simulink model "Project_Sim_Thyr"  (R2022b)
settings: Solver=FixedStepAuto  StartTime=0.0  StopTime=10  FixedStep=0.0001  RelTol=1e-3
libraries: spsVoltageMeasurementLib x6, spsThyristorLib x5, spsGroundLib x3, spsSeriesRLCBranchLib x3, spsControlledVoltageSourceLib x2, spsACVoltageSourceLib x1, spsCurrentMeasurementLib x1, spsDCMachineLib x1, spsDiodeLib x1, spsMeanLib x1, spsMosfetLib x1, spsPWMGeneratorDCDCLib x1
settings Model: Creator=Lenovo  LastModifiedBy=Lenovo

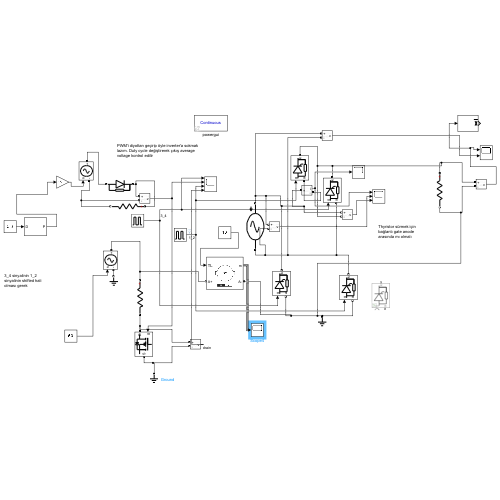
[thumbnail: Simulink's stored preview of the top-level diagram]
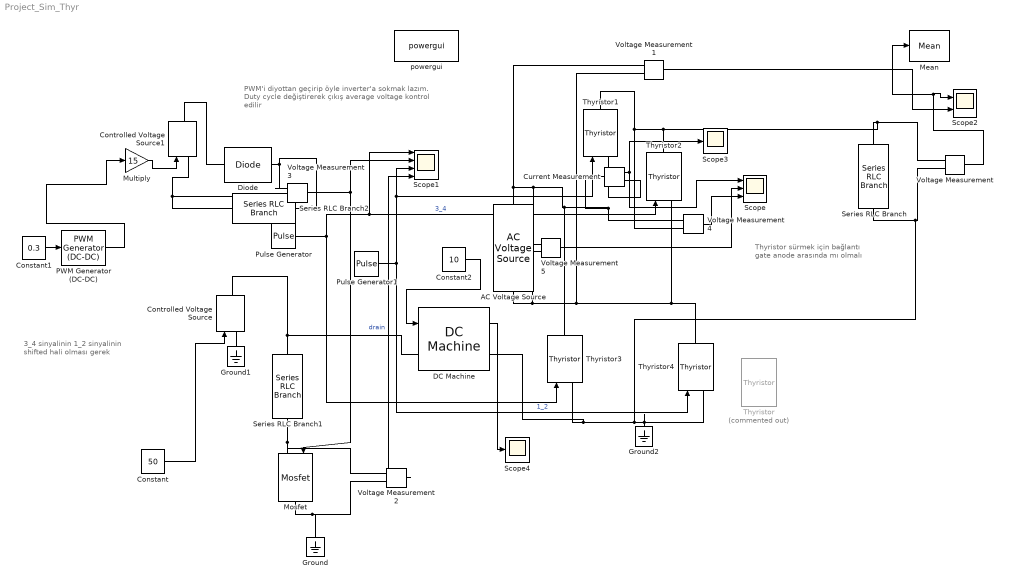
== system Project_Sim_Thyr ==
  note: Thyristor sürmek için bağlantı gate anode arasında mı olmalı
  note: 3_4 sinyalinin 1_2 sinyalinin shifted hali olması gerek
  note: PWM'i diyottan geçirip öyle inverter'a sokmak lazım. Duty cycle değiştirerek çıkış average voltage kontrol edilir
  AC Voltage Source : spsACVoltageSourceLib/AC Voltage Source  Amplitude=230  Phase=0  Frequency=50  SampleTime=0  Measurements=None  BusType=swing  Pref=10e3  Qref=0  Qmin=-inf  Qmax=+inf
  Constant : Constant  Value=50
  Constant1 : Constant  Value=0.3
  Constant2 : Constant  Value=10
  Controlled Voltage Source : spsControlledVoltageSourceLib/Controlled Voltage Source  Initialize=on  Source_Type=DC  Amplitude=15  Phase=0  Frequency=0  Measurements=None
  Controlled Voltage Source1 : spsControlledVoltageSourceLib/Controlled Voltage Source  Initialize=on  Source_Type=DC  Amplitude=0  Phase=0  Frequency=0  Measurements=None
  Current Measurement : spsCurrentMeasurementLib/Current Measurement  PhasorSimulation=off  OutputType=Complex  PSBequivalent=0
  DC Machine : spsDCMachineLib/DC Machine  PresetModel=No  MechanicalLoad=Torque TL  FieldType=Permanent magnet  ShowDetailedParameters=on  MeasurementBus=off  RLa="[ 0.6  0.012]"  RLf="[ 240  120]"  Laf=1.8  MachineConstant=Torque constant (N.m/A)  Ke=1.8  Kt=1.8  J=1  Bm=0  Tf=0  w0=1  Ifinit=1  TsPowergui=0  TsBlock=-1
  Diode : spsDiodeLib/Diode  Ron=0.001  Lon=0  Vf=0.8  IC=0  UseSnubber=0  Rs=500  Cs=250e-9  Measurements=off
  Ground : spsGroundLib/Ground  LConnTagsString=a
  Ground1 : spsGroundLib/Ground  LConnTagsString=a
  Ground2 : spsGroundLib/Ground  LConnTagsString=a
  Mean : spsMeanLib/Mean  Freq=50  Vinit=0  Ts=0
  Mosfet : spsMosfetLib/Mosfet  Ron=0.1  Lon=0  Rd=0.01  Vfd=1  IC=0  Rs=1e5  Cs=inf  Measurements=off
  Multiply : Gain  Gain=15
  PWM Generator (DC-DC) : spsPWMGeneratorDCDCLib/PWM Generator (DC-DC)  Fsw=50  Ts=0
  Pulse Generator : DiscretePulseGenerator  PulseType=Time based  Amplitude=15  Period=0.02  PulseWidth=50  PhaseDelay=0.01+0.02*0.3  VectorParams1D=off
  Pulse Generator1 : DiscretePulseGenerator  PulseType=Time based  Amplitude=15  Period=0.02  PulseWidth=50  PhaseDelay=0.02*0.3
  Scope : Scope  NumInputPorts=3
  Scope1 : Scope  NumInputPorts=4
  Scope2 : Scope  NumInputPorts=2
  Scope3 : Scope
  Scope4 : Scope
  Series RLC Branch : spsSeriesRLCBranchLib/Series RLC Branch  LConnTagsString=__new0  RConnTagsString=__new0  BranchType=R  Resistance=100  Inductance=1e-3  SetiL0=off  InitialCurrent=0  Capacitance=1e-6  Setx0=off  InitialVoltage=0  Measurements=None
  Series RLC Branch1 : spsSeriesRLCBranchLib/Series RLC Branch  LConnTagsString=__new0  RConnTagsString=__new0  BranchType=R  Resistance=10  Inductance=1e-3  SetiL0=off  InitialCurrent=0  Capacitance=1e-6  Setx0=off  InitialVoltage=0  Measurements=None
  Series RLC Branch2 : spsSeriesRLCBranchLib/Series RLC Branch  LConnTagsString=__new0  RConnTagsString=__new0  BranchType=R  Resistance=1000  Inductance=1e-3  SetiL0=off  InitialCurrent=0  Capacitance=1e-6  Setx0=off  InitialVoltage=0  Measurements=None
  Thyristor : spsThyristorLib/Thyristor  Commented=on  Ron=0.001  Lon=0  Vf=50  IC=0  Rs=500  Cs=250e-9  Measurements=off
  Thyristor{1..4} (4 alike) : spsThyristorLib/Thyristor  Ron=1  Lon=0  Vf=5  IC=0  Rs=500  Cs=250e-9  Measurements=off
  Voltage Measurement{,1..5} (6 alike) : spsVoltageMeasurementLib/Voltage Measurement  PhasorSimulation=off  OutputType=Complex  PSBequivalent=0
  powergui : spspowerguiLib/powergui  Priority=1  SimulationMode=Continuous  SampleTime=50e-6  frequency=60  Iterations=50  frequencyindice=0  Pbase=100e6  ErrMax=1e-4  UnitsV=kV  UnitsW=MW  buscounter=0  FunctionMessages=off  echomessages=off  EnableUseOfTLC=off  CurrentSourceSwitches=off  DisableSnubberDevices=off  DisableRonSwitches=off  DisableVfSwitches=off  DisplayEquations=off  AutomaticDiscreteSolvers=off  SolverType=Tustin/Backward Euler (TBE)  Interpol=off  ExternalGateDelay=off  methode=off  Ts=100  x0status=blocks  SPID=on  SwTol=0  HookPort=off  NonlinearTolerance=1e-4  nMaxIteration=100  ContinueOnMaxIteration=off  RestoreLinks=warning  ResistiveCurrentMeasurement=off  Frange=[0:2:500]  Ylog=off  Xlog=on  ShowGrid=off  save=off  variable=ZData  structure=0  ZoomFFT=off  StartTime=0.0  cycles=1  DisplayStyle=1  fundamental=60  FreqAxis=off  MaxFrequency=1000  frequencyindicesteady=1  RmsSteady=1  display=off
  wires:
  Voltage Measurement/1 -> Mean/1, Scope2/1
  Pulse Generator1/1 -> Thyristor4/1, Thyristor1/1, Scope1/3  "1_2"
  Voltage Measurement2/1 -> Scope1/4  "drain"
  Pulse Generator/1 -> Thyristor2/1, Scope1/1, Thyristor3/1  "3_4"
  Constant1/1 -> PWM Generator (DC-DC)/1
  Multiply/1 -> Controlled Voltage Source1/1
  Voltage Measurement3/1 -> Scope1/2, Mosfet/1
  PWM Generator (DC-DC)/1 -> Multiply/1
  Voltage Measurement1/1 -> Scope2/2
  Voltage Measurement4/1 -> Scope/3
  Voltage Measurement5/1 -> Scope/2
  Current Measurement/1 -> Scope/1, Scope3/1
  Constant2/1 -> DC Machine/1
  DC Machine/1 -> Scope4/1
  Constant/1 -> Controlled Voltage Source/1
  connections:
  Series RLC Branch/LConn1 -- Voltage Measurement4/LConn2 -- Thyristor1/RConn1 -- Thyristor2/RConn1 -- Voltage Measurement/LConn1
  Voltage Measurement1/LConn1 -- Voltage Measurement5/LConn1 -- Current Measurement/LConn1 -- Voltage Measurement4/LConn1 -- Thyristor3/RConn1 -- AC Voltage Source/RConn1
  Mosfet/RConn1 -- Voltage Measurement2/LConn2 -- Ground/LConn1
  Thyristor4/RConn1 -- Thyristor2/LConn1 -- Voltage Measurement1/LConn2 -- Voltage Measurement5/LConn2 -- AC Voltage Source/LConn1
  Mosfet/LConn1 -- Voltage Measurement2/LConn1 -- Series RLC Branch1/RConn1
  Controlled Voltage Source/RConn1 -- DC Machine/LConn1 -- Series RLC Branch1/LConn1
  Controlled Voltage Source1/RConn1 -- Diode/LConn1
  Controlled Voltage Source1/LConn1 -- Voltage Measurement3/LConn2 -- Series RLC Branch2/RConn1
  Series RLC Branch2/LConn1 -- Voltage Measurement3/LConn1 -- Diode/RConn1
  Ground1/LConn1 -- Controlled Voltage Source/LConn1
  Series RLC Branch/RConn1 -- Ground2/LConn1 -- Thyristor4/LConn1 -- DC Machine/RConn1 -- Thyristor3/LConn1 -- Voltage Measurement/LConn2
  Current Measurement/RConn1 -- Thyristor1/LConn1
